simulink model "recursive_ssm_update"  (R2020a)
settings: Solver=FixedStepAuto  StartTime=1939  StopTime=1970  FixedStep=1  RelTol=1e-3
settings Model: Creator=tyoshida  LastModifiedBy=tyoshida

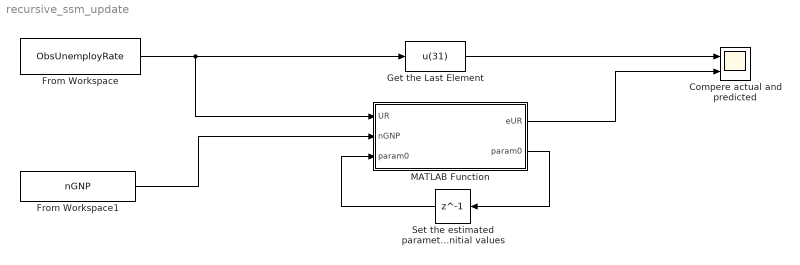
== system recursive_ssm_update ==
  Compere actual and predicted : Scope  NumInputPorts=2
  From Workspace : FromWorkspace  VariableName=ObsUnemployRate
  From Workspace1 : FromWorkspace  VariableName=nGNP
  Get the Last Element : Fcn  Expr=u(31)
  MATLAB Function : MATLAB Function  TreatAsAtomicUnit=on
  Set the estimated parameters as the next iteration of their initial values : Delay  DelayLength=1  InitialCondition=[0.5; 0.1; -20]
  wires:
  From Workspace/1 -> Get the Last Element/1, MATLAB Function/1(UR)
  From Workspace1/1 -> MATLAB Function/2(nGNP)
  MATLAB Function/1(eUR) -> Compere actual and predicted/2
  MATLAB Function/2(param0) -> Set the estimated parameters as the next iteration of their initial values/1
  Set the estimated parameters as the next iteration of their initial values/1 -> MATLAB Function/3("param0 ")
  Get the Last Element/1 -> Compere actual and predicted/1

== matlab function recursive_ssm_update/MATLAB Function ==
  data: UR input; eUR output; nGNP input; param0 output; param0 input
function [eUR, param0]  = SSM_Predictor(UR, nGNP, param0)

yhat = 0; %#ok<NASGU> % WA because the analyzer cannot identify this data type for code generation
% param0 = [0.5; 0.1; -20];

Z = diff(log(nGNP));
y = diff(UR);

coder.extrinsic('my_predict_fcn'); % declare extrinsic functions for code generation
[yhat, param0] = my_predict_fcn(y, Z, param0);

eUR = yhat + UR(end);

% MATLAB function doesn't support function handle
%{
Mdl = ssm(@(c)rwAR2ParamMap(c,y,Z));
[Mdl, param0] = estimate(Mdl, y, param0, 'Display', 'off');
yhat = forecast(Mdl, 1, y,'Predictors0',Z,'PredictorsF',Z(end),'Beta',param0(end));
eUR = UR(end) + yhat;
%}

end
